simulink model "simulink_optimal_servo_R2023a"  (R2023a)
settings: Solver=ode4  StartTime=0.0  StopTime=10.0  FixedStep=0.01  RelTol=1e-3  EnableMultiTasking=on
values from neighbouring files (symbols this model uses):
  A = [  0  1 ... (first row only)    [optimal_care.m]    (also in optimal_hamilton.m; optimal_hamilton2.m; optimal_lqr.m; optimal_servo.m = [ 0  1  0  0)
  B = [ 0 ... (first row only)    [optimal_care.m]    (also in optimal_hamilton.m; optimal_hamilton2.m; optimal_lqr.m; optimal_servo.m)
  C = [ 0  0  1  0 ]    [optimal_servo.m]
  Fa = [ -K+2*G*inv(P22)*P12'  1 ]*inv(M0)*[ zeros(4,1); 1 ]    [optimal_servo.m]
  Fb = - 2*G*inv(P22)*P12'    [optimal_servo.m]
  G = - inv(Re)*B'*P12    [optimal_servo.m]
  K = - inv(R)*B'*P    [optimal_care.m]    (also in optimal_lqr.m = - lqr(A,B,Q,R); optimal_servo.m = - inv(Re)*B'*P11; symb_riccati.m = double(K))
  x0 = [ 1  0 ]'    [run_simulink_lqr.m]    (also in run_simulink_optimal_servo.m = [ 0  0  0.25  0 ]')
settings Model: Creator=kawata  LastModifiedBy=kawata
settings SolverCC: AlgebraicLoopSolver=TrustRegion
settings DataIOCC: LimitDataPoints=on  SaveFormat=Array  SignalLoggingSaveFormat=ModelDataLogs  ReturnWorkspaceOutputs=off
settings OptimizationCC: ExpressionDepthLimit=2147483647  LifeSpan=inf
settings DebuggingCC: UnderspecifiedInitializationDetection=Classic  MergeDetectMultiDrivingBlocksExec=none  SolverPrmCheckMsg=warning  FcnCallInpInsideContextMsg=warning  UnconnectedInputMsg=warning  UnconnectedOutputMsg=warning  UnconnectedLineMsg=warning  StateNameClashWarn=warning  SFUnexpectedBacktrackingDiag=warning  SFNoUnconditionalDefaultTransitionDiag=warning  SFExecutionAtInitializationDiag=none  ArithmeticOperatorsInVariantConditions=warning
settings HardwareCC: ProdBitPerPointer=32  ProdBitPerSizeT=32  ProdBitPerPtrDiffT=32  ProdLargestAtomicFloat=None  ProdIntDivRoundTo=Undefined  ProdEndianess=Unspecified  ProdWordSize=32  ProdHWDeviceType=32-bit Generic
settings ModelReferenceCC: EnableRefExpFcnMdlSchedulingChecks=on  PropagateSignalLabelsOutOfModel=off
settings SFSimCC: SimUseLocalCustomCode=off  CustomCodeUndefinedFunction=UseInterfaceOnly
settings RTWCC: RTWUseLocalCustomCode=off
settings CodeAppCC: StateflowObjectComments=on
settings GRTTargetCC: TargetLangStandard=C89/C90 (ANSI)  CombineOutputUpdateFcns=off  GRTInterface=on
settings ConfigComp: CovMetricSettings=dw  CovSaveCumulativeToWorkspaceVar=on  CovSaveSingleToWorkspaceVar=on  CovExternalEMLEnable=off

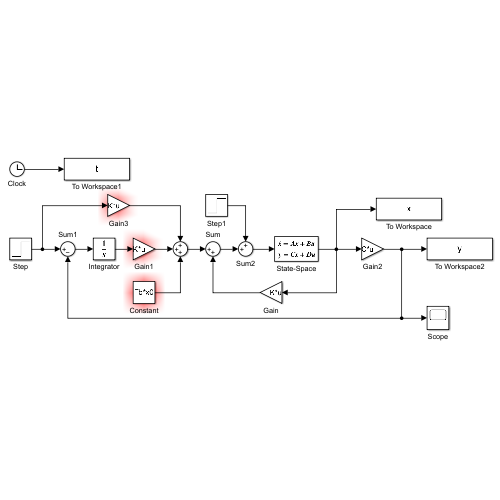
[thumbnail: Simulink's stored preview of the top-level diagram]
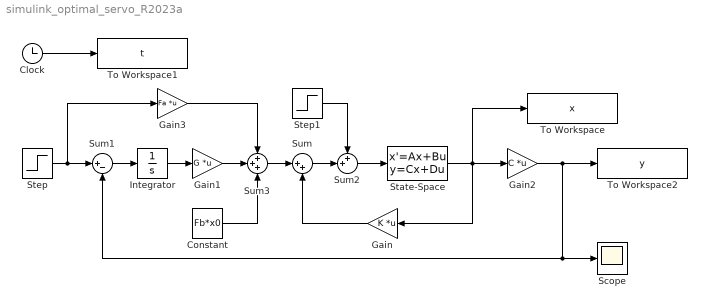
== system simulink_optimal_servo_R2023a ==
  Clock : Clock
  Constant : Constant  Value=Fb*x0
  Gain : Gain  Gain=K  Multiplication=Matrix(K*u)
  Gain1 : Gain  Gain=G  Multiplication=Matrix(K*u)
  Gain2 : Gain  Gain=C  Multiplication=Matrix(K*u)
  Gain3 : Gain  Gain=Fa  Multiplication=Matrix(K*u)
  Integrator : Integrator
  Scope : Scope
  State-Space : StateSpace  A=A  B=B  C=eye(4)  D=zeros(4,1)  InitialCondition=x0
  Step : Step  Time=0  SampleTime=0
  Step1 : Step  Time=5  SampleTime=0
  Sum : Sum  Inputs=|++  InputSameDT=on  SaturateOnIntegerOverflow=on  OutDataTypeStr=Inherit: Same as first input
  Sum1 : Sum  Inputs=|+-  InputSameDT=on  SaturateOnIntegerOverflow=on  OutDataTypeStr=Inherit: Same as first input
  Sum2 : Sum  Inputs=++|  InputSameDT=on  SaturateOnIntegerOverflow=on  OutDataTypeStr=Inherit: Same as first input
  Sum3 : Sum  Inputs=+++  InputSameDT=on  SaturateOnIntegerOverflow=on  OutDataTypeStr=Inherit: Same as first input
  To Workspace : ToWorkspace  VariableName=x  SampleTime=-1
  To Workspace1 : ToWorkspace  VariableName=t  SampleTime=-1
  To Workspace2 : ToWorkspace  VariableName=y  SampleTime=-1
  wires:
  State-Space/1 -> To Workspace/1, Gain/1, Gain2/1
  Clock/1 -> To Workspace1/1
  Sum1/1 -> Integrator/1
  Gain2/1 -> To Workspace2/1, Sum1/2, Scope/1
  Step/1 -> Gain3/1, Sum1/1
  Integrator/1 -> Gain1/1
  Gain/1 -> Sum/2
  Sum/1 -> Sum2/2
  Sum2/1 -> State-Space/1
  Step1/1 -> Sum2/1
  Constant/1 -> Sum3/3
  Gain1/1 -> Sum3/2
  Sum3/1 -> Sum/1
  Gain3/1 -> Sum3/1
